simulink model "sampleModel1732"  (R2023a)
settings: Solver=VariableStepAuto  StartTime=0.0  StopTime=10.0  RelTol=1e-3
libraries: hdlsllib x6, simulink x1
settings Model: Creator=user1  LastModifiedBy=user1

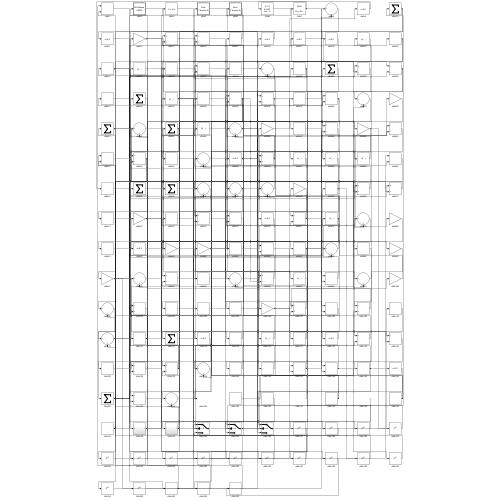
[thumbnail: Simulink's stored preview of the top-level diagram]
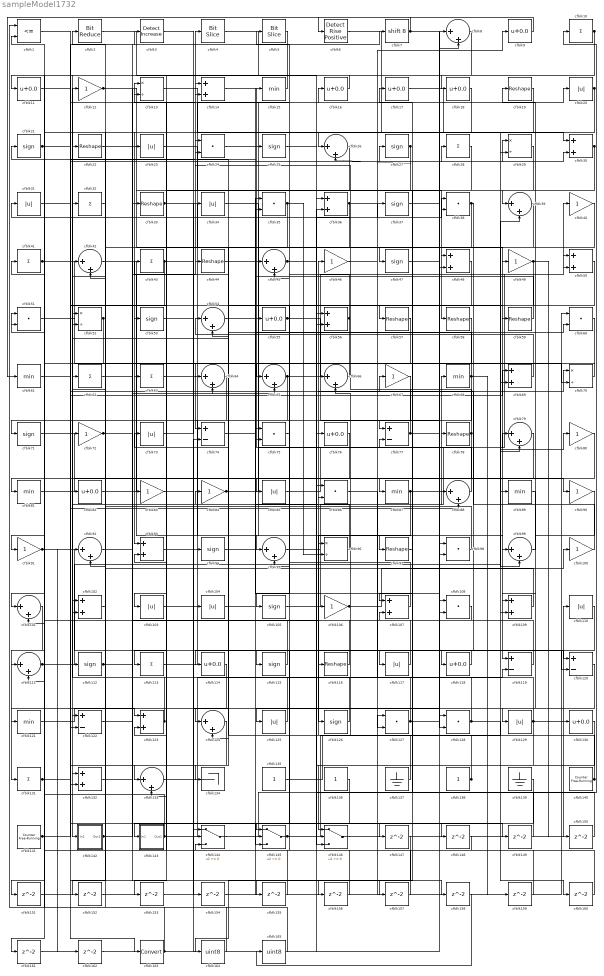
== system sampleModel1732 ==
  cfblk1 : RelationalOperator  Operator=<=  OutDataTypeStr=boolean  InputSameDT=off
  cfblk{10,28,32,41,43,62..63,113,131} (9 alike) : Sum  Inputs=+
  cfblk{12,40,46,49,67,72,80,83..84,90..91,100,106} (13 alike) : Gain
  cfblk{8,26,39,42,45,54,64..66,79,88,92,95,99,101,111,124,133} (18 alike) : Sum  Inputs=|++
  cfblk{14,30,36,48,50,56,69,93,102,107,109,123,132} (13 alike) : Sum
  cfblk{20,23,31,34,73,85,103..104,110,117,125,129} (12 alike) : Abs  SaturateOnIntegerOverflow=off
  cfblk{21,25,27,37,47,53,71,94,105,112,115,126} (12 alike) : Signum
  cfblk{24,35,38,51,60,75,86,98,108,127..128} (11 alike) : DotProduct  OutDataTypeStr=Inherit: Inherit via internal rule
  cfblk{9,11,16..18,55,76,82,114,118,130} (11 alike) : Bias  Bias=0.0  SaturateOnIntegerOverflow=off
  cfblk{19,22,33,44,57..59,78,97,116} (10 alike) : Reshape
  cfblk{74,77,119..120,122} (5 alike) : Sum  Inputs=+-
  cfblk{15,61,68,81,87,89,121} (7 alike) : MinMax
  cfblk{13,29,52,70,96} (5 alike) : Product  Inputs=*/  RndMeth=Zero  SaturateOnIntegerOverflow=on
  cfblk134 : Terminator
  cfblk135 : Constant  SampleTime=-1
  cfblk136 : Constant  SampleTime=-1
  cfblk137 : Ground
  cfblk138 : Constant  SampleTime=-1
  cfblk139 : Ground
  cfblk140 : hdlsllib/Sources/Counter Free-Running  NumBits=16  tsamp=-1
  cfblk141 : hdlsllib/Sources/Counter Free-Running  NumBits=16  tsamp=-1
  cfblk142 : Subsystem
      settings: LibrarySourceBlock=|
      | hdlsllib/Ports &
      | Subsystems/Subsystem
  cfblk143 : Subsystem
      settings: LibrarySourceBlock=|
      | hdlsllib/Ports &
      | Subsystems/Subsystem
  cfblk144 : Switch  SaturateOnIntegerOverflow=off  InputSameDT=off
  cfblk145 : Switch  SaturateOnIntegerOverflow=off  InputSameDT=off
  cfblk146 : Switch  SaturateOnIntegerOverflow=off  InputSameDT=off
  cfblk{147..162} (16 alike) : Delay  SampleTime=1
  cfblk163 : DataTypeConversion  SaturateOnIntegerOverflow=off  RndMeth=Floor
  cfblk164 : DataTypeConversion  OutDataTypeStr=uint8  SaturateOnIntegerOverflow=off  RndMeth=Floor
  cfblk165 : DataTypeConversion  OutDataTypeStr=uint8  SaturateOnIntegerOverflow=off  RndMeth=Floor
  cfblk2 : hdlsllib/Logic and Bit Operations/Bit Reduce  mode=AND
  cfblk3 : simulink/Logic and Bit Operations/Detect Increase  vinit=0.0  OutDataTypeStr=boolean
      settings: LibrarySourceBlock=|
      | hdlsllib/Logic and Bit
      | Operations/Detect
      | Increase
  cfblk4 : hdlsllib/Logic and Bit Operations/Bit Slice  lidx=7  ridx=0
  cfblk5 : hdlsllib/Logic and Bit Operations/Bit Slice  lidx=7  ridx=0
  cfblk6 : hdlsllib/Logic and Bit Operations/Detect Rise Positive  vinit=0  OutDataTypeStr=boolean
  cfblk7 : ArithShift  BitShiftNumber=8
  wires:
  cfblk140/1 -> cfblk46/1, cfblk52/2
  cfblk22/1 -> cfblk119/1
  cfblk84/1 -> cfblk28/1, cfblk78/1
  cfblk88/1 -> cfblk15/1
  cfblk64/1 -> cfblk95/1
  cfblk93/1 -> cfblk16/1
  cfblk107/1 -> cfblk13/1
  cfblk6/1 -> cfblk30/1
  cfblk16/1 -> cfblk142/1(In1)
  cfblk54/1 -> cfblk20/1
  cfblk144/1 -> cfblk10/1
  cfblk63/1 -> cfblk25/1
  cfblk75/1 -> cfblk105/1
  cfblk18/1 -> cfblk93/1
  cfblk29/1 -> cfblk39/1
  cfblk112/1 -> cfblk33/1, cfblk42/1
  cfblk12/1 -> cfblk58/1, cfblk120/2
  cfblk15/1 -> cfblk11/1
  cfblk4/1 -> cfblk36/1
  cfblk96/1 -> cfblk12/1
  cfblk14/1 -> cfblk99/1
  cfblk113/1 -> cfblk67/1
  cfblk118/1 -> cfblk114/1
  cfblk47/1 -> cfblk98/1
  cfblk72/1 -> cfblk64/2, cfblk156/1
  cfblk42/1 -> cfblk126/1
  cfblk126/1 -> cfblk13/2
  cfblk141/1 -> cfblk70/1, cfblk101/2
  cfblk2/1 -> cfblk76/1
  cfblk34/1 -> cfblk128/1
  cfblk91/1 -> cfblk115/1, cfblk24/1, cfblk162/1
  cfblk67/1 -> cfblk77/1
  cfblk101/1 -> cfblk131/1
  cfblk33/1 -> cfblk49/1, cfblk96/1, cfblk128/2
  cfblk7/1 -> cfblk61/1, cfblk69/2
  cfblk114/1 -> cfblk121/1
  cfblk133/1 -> cfblk37/1
  cfblk128/1 -> cfblk32/1, cfblk160/1
  cfblk138/1 -> cfblk43/1, cfblk66/2
  cfblk90/1 -> cfblk129/1
  cfblk82/1 -> cfblk4/1
  cfblk89/1 -> cfblk109/1
  cfblk119/1 -> cfblk75/1
  cfblk65/1 -> cfblk8/1, cfblk133/2
  cfblk17/1 -> cfblk99/2
  cfblk79/1 -> cfblk132/1
  cfblk20/1 -> cfblk26/1, cfblk71/1
  cfblk117/1 -> cfblk5/1
  cfblk35/1 -> cfblk103/1, cfblk53/1, cfblk52/1, cfblk96/2
  cfblk98/1 -> cfblk22/1
  cfblk124/1 -> cfblk132/2
  cfblk92/1 -> cfblk44/1
  cfblk38/1 -> cfblk118/1, cfblk42/2
  cfblk26/1 -> cfblk83/1
  cfblk106/1 -> cfblk100/1, cfblk120/1
  cfblk121/1 -> cfblk123/1
  cfblk145/1 -> cfblk109/2, cfblk119/2
  cfblk116/1 -> cfblk92/1
  cfblk135/1 -> cfblk39/2
  cfblk59/1 -> cfblk45/1
  cfblk81/1 -> cfblk87/1
  cfblk111/1 -> cfblk80/1, cfblk14/2
  cfblk146/1 -> cfblk110/1
  cfblk110/1 -> cfblk145/1
  cfblk37/1 -> cfblk8/2
  cfblk85/1 -> cfblk40/1
  cfblk76/1 -> cfblk81/1
  cfblk10/1 -> cfblk113/1, cfblk133/1
  cfblk9/1 -> cfblk6/1
  cfblk122/1 -> cfblk7/1
  cfblk49/1 -> cfblk124/2, cfblk150/1
  cfblk69/1 -> cfblk54/1
  cfblk109/1 -> cfblk62/1
  cfblk131/1 -> cfblk29/1, cfblk3/1, cfblk145/3, cfblk69/1
  cfblk143/1(Out1) -> cfblk55/1, cfblk41/1
  cfblk73/1 -> cfblk34/1
  cfblk86/1 -> cfblk127/2
  cfblk104/1 -> cfblk75/2
  cfblk56/1 -> cfblk74/1, cfblk31/1, cfblk14/1
  cfblk127/1 -> cfblk112/1, cfblk50/1
  cfblk36/1 -> cfblk134/1, cfblk38/2
  cfblk125/1 -> cfblk84/1
  cfblk68/1 -> cfblk21/1, cfblk111/2, cfblk159/1
  cfblk137/1 -> cfblk73/1
  cfblk5/1 -> cfblk91/1
  cfblk77/1 -> cfblk98/2, cfblk35/2
  cfblk48/1 -> cfblk124/1
  cfblk60/1 -> cfblk117/1
  cfblk55/1 -> cfblk108/1, cfblk38/1
  cfblk1/1 -> cfblk163/1
  cfblk24/1 -> cfblk108/2
  cfblk31/1 -> cfblk27/1
  cfblk52/1 -> cfblk101/1, cfblk161/1
  cfblk44/1 -> cfblk47/1
  cfblk23/1 -> cfblk86/1
  cfblk123/1 -> cfblk102/1, cfblk2/1
  cfblk45/1 -> cfblk48/1, cfblk97/1
  cfblk30/1 -> cfblk107/1, cfblk56/2
  cfblk142/1(Out1) -> cfblk23/1, cfblk106/1
  cfblk99/1 -> cfblk19/1
  cfblk94/1 -> cfblk86/2
  cfblk51/1 -> cfblk144/2
  cfblk115/1 -> cfblk51/1
  cfblk71/1 -> cfblk90/1
  cfblk100/1 -> cfblk66/1
  cfblk66/1 -> cfblk64/1
  cfblk105/1 -> cfblk79/1
  cfblk57/1 -> cfblk111/1
  cfblk32/1 -> cfblk72/1
  cfblk61/1 -> cfblk30/2
  cfblk78/1 -> cfblk24/2, cfblk85/1, cfblk153/1
  cfblk21/1 -> cfblk59/1, cfblk88/2
  cfblk129/1 -> cfblk17/1, cfblk130/1, cfblk146/2
  cfblk46/1 -> cfblk9/1
  cfblk25/1 -> cfblk70/2
  cfblk136/1 -> cfblk145/2
  cfblk87/1 -> cfblk116/1, cfblk88/1, cfblk50/2
  cfblk139/1 -> cfblk143/1(In1)
  cfblk74/1 -> cfblk60/2
  cfblk95/1 -> cfblk68/1
  cfblk70/1 -> cfblk65/1
  cfblk3/1 -> cfblk94/1
  cfblk28/1 -> cfblk57/1
  cfblk108/1 -> cfblk107/2
  cfblk53/1 -> cfblk65/2
  cfblk8/1 -> cfblk18/1
  cfblk40/1 -> cfblk54/2
  cfblk80/1 -> cfblk92/2
  cfblk43/1 -> cfblk104/1, cfblk122/2, cfblk63/1
  cfblk41/1 -> cfblk79/2, cfblk89/1
  cfblk130/1 -> cfblk146/1
  cfblk13/1 -> cfblk29/2
  cfblk50/1 -> cfblk95/2
  cfblk102/1 -> cfblk122/1
  cfblk120/1 -> cfblk125/1
  cfblk27/1 -> cfblk26/2, cfblk146/3
  cfblk39/1 -> cfblk147/1
  cfblk132/1 -> cfblk148/1
  cfblk148/1 -> cfblk144/3
  cfblk103/1 -> cfblk149/1
  cfblk149/1 -> cfblk56/1
  cfblk150/1 -> cfblk77/2
  cfblk58/1 -> cfblk151/1
  cfblk151/1 -> cfblk127/1
  cfblk19/1 -> cfblk152/1
  cfblk152/1 -> cfblk102/2
  cfblk153/1 -> cfblk60/1
  cfblk83/1 -> cfblk154/1
  cfblk154/1 -> cfblk35/1
  cfblk62/1 -> cfblk155/1
  cfblk155/1 -> cfblk144/1
  cfblk156/1 -> cfblk93/2
  cfblk97/1 -> cfblk157/1
  cfblk157/1 -> cfblk45/2
  cfblk11/1 -> cfblk158/1
  cfblk159/1 -> cfblk123/2
  cfblk160/1 -> cfblk51/2
  cfblk161/1 -> cfblk74/2
  cfblk162/1 -> cfblk36/2
  cfblk163/1 -> cfblk48/2, cfblk82/1
  cfblk147/1 -> cfblk164/1
  cfblk164/1 -> cfblk1/1
  cfblk158/1 -> cfblk165/1
  cfblk165/1 -> cfblk1/2

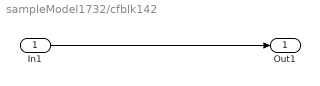
== system sampleModel1732/cfblk142 ==
  In1 : Inport
  Out1 : Outport
  wires:
  In1/1 -> Out1/1

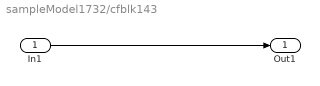
== system sampleModel1732/cfblk143 ==
  In1 : Inport
  Out1 : Outport
  wires:
  In1/1 -> Out1/1
